simulink model "Simulation_DC_Estimate"  (R2021a)
settings: Solver=ode5  StartTime=ti  StopTime=tf  FixedStep=Ts/40  RelTol=1e-3
undefined symbols (not defined in the file): A_real, B_real, Cx_real, Dx_real, f, IC, Noise, torque, u0, umax
libraries: simulink x1
settings Model: Creator=perruquetti  LastModifiedBy=perruquetti
settings SolverCC: AlgebraicLoopSolver=TrustRegion
settings DataIOCC: ReturnWorkspaceOutputs=off
settings DebuggingCC: SFMachineParentedDataDiag=warning  ArithmeticOperatorsInVariantConditions=warning
settings SFSimCC: SimUseLocalCustomCode=off  CustomCodeUndefinedFunction=UseInterfaceOnly
settings RTWCC: RTWUseLocalCustomCode=off

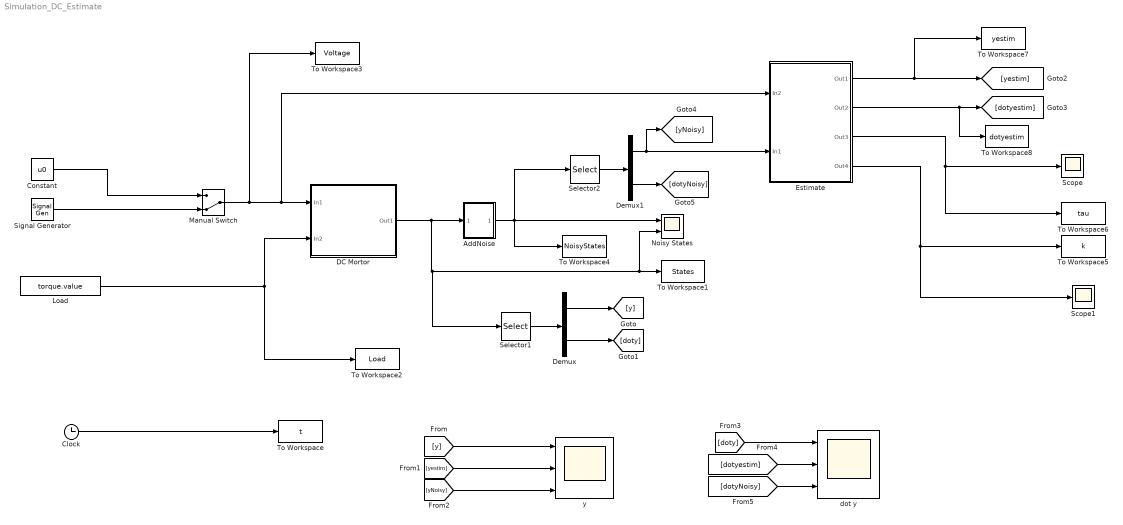
== system Simulation_DC_Estimate ==
  AddNoise : Subsystem
  Clock : Clock
  Constant : Constant  Value=u0
  DC Mortor : Subsystem
      mask Display: image('motor2.png');
  Demux : Demux  Outputs=2
  Demux1 : Demux  Outputs=2
  Estimate : Subsystem
  Load : Constant  Value=torque.value
  Manual Switch : ManualSwitch  CurrentSetting=0
  Noisy States : Scope  NumInputPorts=2
  Scope : Scope
  Scope1 : Scope
  Selector1 : Selector  InputPortWidth=3  IndexOptions=Index vector (dialog)  Indices=[1 2]  OutputSizes=1
  Selector2 : Selector  InputPortWidth=3  IndexOptions=Index vector (dialog)  Indices=[1 2]  OutputSizes=1
  Signal Generator : SignalGenerator  Amplitude=u0  Frequency=f  Units=rad/sec
  To Workspace : ToWorkspace  VariableName=t  SampleTime=-1
  To Workspace1 : ToWorkspace  VariableName=States  SampleTime=-1
  To Workspace2 : ToWorkspace  VariableName=Load  SampleTime=-1
  To Workspace3 : ToWorkspace  VariableName=Voltage  SampleTime=-1
  To Workspace4 : ToWorkspace  VariableName=NoisyStates  SampleTime=-1
  To Workspace5 : ToWorkspace  VariableName=k  SampleTime=-1
  To Workspace6 : ToWorkspace  VariableName=tau  SampleTime=-1
  To Workspace7 : ToWorkspace  VariableName=yestim  SampleTime=-1
  To Workspace8 : ToWorkspace  VariableName=dotyestim  SampleTime=-1
  dot y : Scope  NumInputPorts=3
  y : Scope  NumInputPorts=3
  wires:
  Clock/1 -> To Workspace/1
  DC Mortor/1(Out1) -> Selector1/1, Noisy States/2, To Workspace1/1, AddNoise/1(In1)
  Load/1 -> DC Mortor/2(In2), To Workspace2/1
  Constant/1 -> Manual Switch/1
  Signal Generator/1 -> Manual Switch/2
  Manual Switch/1 -> To Workspace3/1, Estimate/1(In2), DC Mortor/1(In1)
  Estimate/3(Out3) -> To Workspace6/1, Scope/1
  Estimate/4(Out4) -> Scope1/1, To Workspace5/1
  Selector1/1 -> Demux/1
  Demux/1 -> [y]
  Demux/2 -> [doty]
  Estimate/1(Out1) -> To Workspace7/1, [yestim]
  Estimate/2(Out2) -> To Workspace8/1, [dotyestim]
  Selector2/1 -> Demux1/1
  AddNoise/1(Out1) -> Selector2/1, Noisy States/1, To Workspace4/1
  Demux1/1 -> [yNoisy], Estimate/2(In1)
  Demux1/2 -> [dotyNoisy]
  [yNoisy] -> y/3
  [dotyNoisy] -> dot y/3
  [doty] -> dot y/1
  [yestim] -> y/2
  [y] -> y/1
  [dotyestim] -> dot y/2

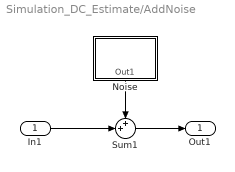
== system Simulation_DC_Estimate/AddNoise ==
  In1 : Inport
  Noise : Subsystem
  Sum1 : Sum  Inputs=++|
  Out1 : Outport
  wires:
  In1/1 -> Sum1/2
  Sum1/1 -> Out1/1
  Noise/1(Out1) -> Sum1/1

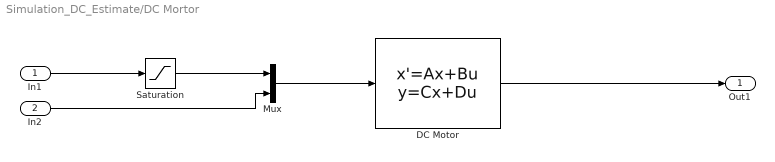
== system Simulation_DC_Estimate/DC Mortor ==
  In1 : Inport
  In2 : Inport  Port=2
  DC Motor : StateSpace  A=A_real  B=B_real  C=Cx_real  D=Dx_real  InitialCondition=IC.state
  Mux : Mux  Inputs=2
  Saturation : Saturate  UpperLimit=umax  LowerLimit=-umax
  Out1 : Outport  VectorParamsAs1DForOutWhenUnconnected=off
  wires:
  DC Motor/1 -> Out1/1
  In1/1 -> Saturation/1
  Saturation/1 -> Mux/1
  Mux/1 -> DC Motor/1
  In2/1 -> Mux/2

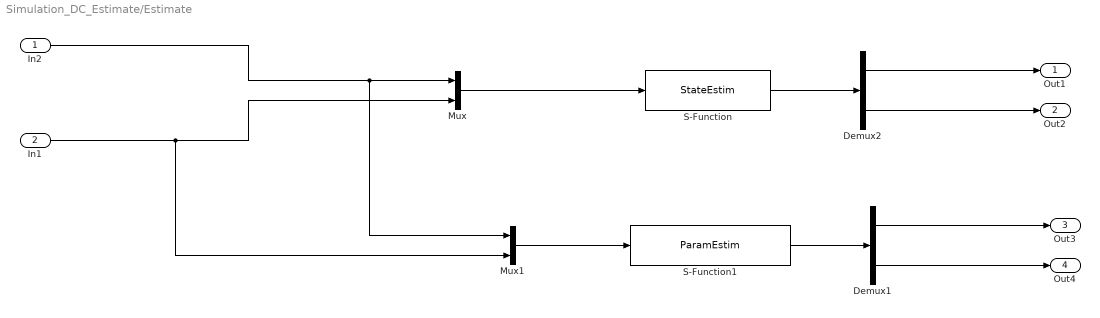
== system Simulation_DC_Estimate/Estimate ==
  In2 : Inport
  In1 : Inport  Port=2
  Demux1 : Demux  Outputs=2
  Demux2 : Demux  Outputs=2
  Mux : Mux  Inputs=2
  Mux1 : Mux  Inputs=2
  S-Function : S-Function  FunctionName=StateEstim  SFunctionDeploymentMode=off  EnableBusSupport=off
  S-Function1 : S-Function  FunctionName=ParamEstim  SFunctionDeploymentMode=off  EnableBusSupport=off
  Out1 : Outport
  Out2 : Outport  Port=2
  Out3 : Outport  Port=3
  Out4 : Outport  Port=4
  wires:
  In2/1 -> Mux1/1, Mux/1
  In1/1 -> Mux1/2, Mux/2
  Mux/1 -> S-Function/1
  Demux2/1 -> Out1/1
  Demux2/2 -> Out2/1
  S-Function/1 -> Demux2/1
  S-Function1/1 -> Demux1/1
  Demux1/1 -> Out3/1
  Demux1/2 -> Out4/1
  Mux1/1 -> S-Function1/1

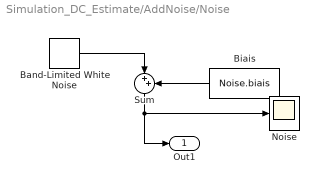
== system Simulation_DC_Estimate/AddNoise/Noise ==
  Band-Limited White Noise : simulink/Sources/Band-Limited White Noise  Cov=Noise.power  Ts=Noise.sampling  seed=Noise.seed
  Biais : Constant  Value=Noise.biais
  Noise : Scope
  Sum : Sum  Inputs=|++
  Out1 : Outport
  wires:
  Sum/1 -> Out1/1, Noise/1
  Biais/1 -> Sum/2
  Band-Limited White Noise/1 -> Sum/1
